simulink model "simulink_ON_OFF"  (R2024a)
settings: Solver=VariableStepAuto  StartTime=0.0  StopTime=20  RelTol=1e-3
settings Model: Creator=Monsty  LastModifiedBy=Monsty

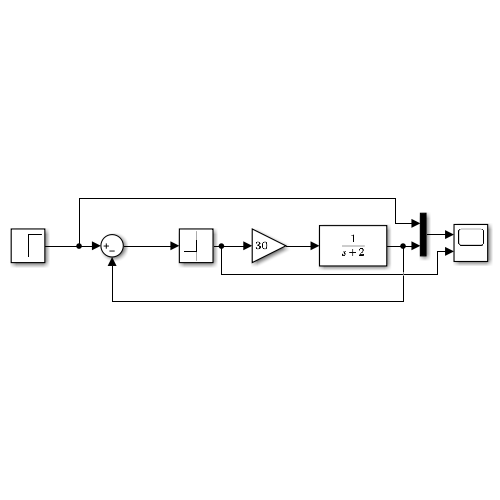
[thumbnail: Simulink's stored preview of the top-level diagram]
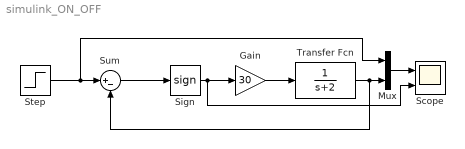
== system simulink_ON_OFF ==
  Gain : Gain  Gain=30
  Mux : Mux  Inputs=2
  Scope : Scope  NumInputPorts=2
  Sign : Signum  ZeroCross=off
  Step : Step  Time=10  Before=1  After=2  SampleTime=0
  Sum : Sum  Inputs=|+-
  Transfer Fcn : TransferFcn  Denominator=[1 2]
  wires:
  Sum/1 -> Sign/1
  Gain/1 -> Transfer Fcn/1
  Mux/1 -> Scope/1
  Step/1 -> Mux/1, Sum/1
  Transfer Fcn/1 -> Sum/2, Mux/2
  Sign/1 -> Scope/2, Gain/1
